simulink model "AE_BoltEV_LMDI"  (R2026a)
settings: Solver=ode23t  StartTime=0  StopTime=1800  FixedStep=Ts  MaxStep=0.01  EnableMultiTasking=on
InitFcn:
  | AE_BoltEV_LMDI_Params;
undefined symbols (not defined in the file): id_map, iq_map, Is_map, n_loss_bp, P, P_cu_map, P_iron_map, T_loss_bp, Tmax, V_oc
libraries: nesl_utility x14, fl_lib x12, autolibshared x2, sdl_lib x2, autolibmappedmotor x1, sl_discontinuities x1
(part 1 of 3)
CloseFcn:
  | try,close(h1_IPMSMTorqueBasedLoad),end
  | clear h1_IPMSMTorqueBasedLoad
  | 
  | clear simlog_IPMSMTorqueBasedLoad
  | clear logsout_IPMSMTorqueBasedLoad
Description:
  | IPMSM Torque-Based Load Control
settings Model: SimulationMode=accelerator  Creator=The MathWorks, Inc.  LastModifiedBy=fsk
settings DataIOCC: Decimation=100  MaxDataPoints=0  OutputTimes=0:0.1:1800  LoggingFileName=Results/paperA_sim_logsout.mat
settings SimscapeCC: SimscapeNormalizeSystem=off  SimscapeNominalValues="[{\"value\":\"1\",\"unit\":\"A\"},{\"value\":\"1\",\"unit\":\"bar\"},{\"value\":\"1\",\"unit\":\"cm^2\"},{\"value\":\"1\",\"unit\":\"cm^3/s\"},{\"value\":\"1\",\"unit\":\"kJ/kg\"},{\"value\":\"1\",\"unit\":\"kW\"},{\"value\":\"1\",\"unit\":\"l\"},{\"value\":\"1\",\"unit\":\"N\"},{\"value\":\"1\",\"unit\":\"N*m\"},{\"value\":\"1\",\"unit\":\"V\"}]"  SimscapeLogType=none  SimscapeLogSimulationStatistics=on  SimscapeLogToSDI=on  SimscapeLogName=simlog_TeslaBEV  SimscapeLogDecimation=50.0  SimscapeLogDataHistory=210000.0

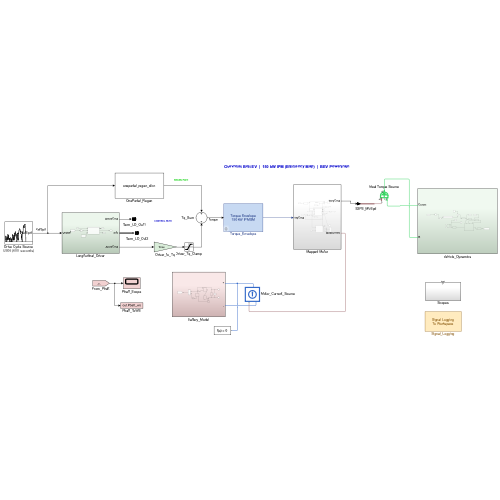
[thumbnail: Simulink's stored preview of the top-level diagram]
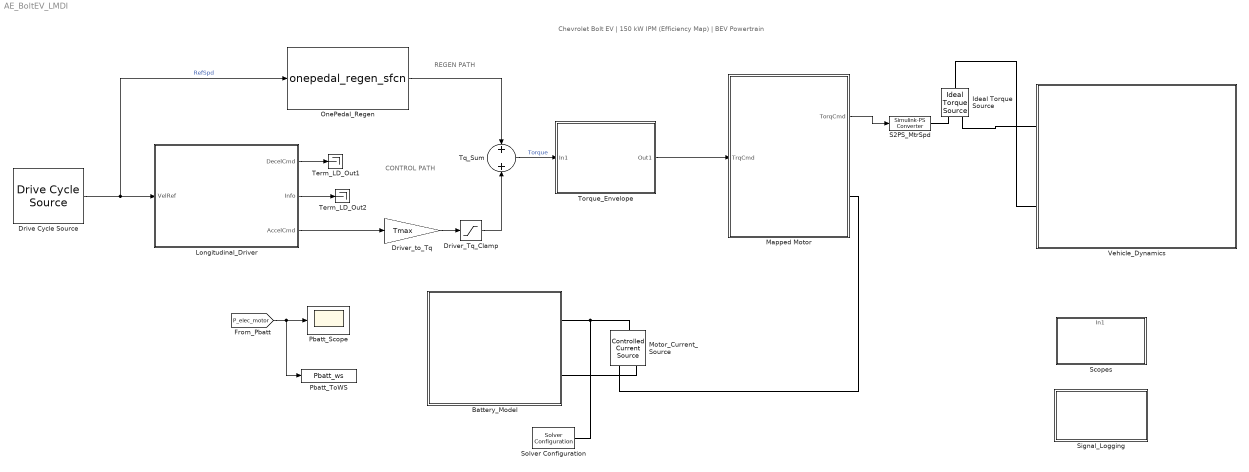
== system AE_BoltEV_LMDI ==
  note: Chevrolet Bolt EV | 150 kW IPM (Efficiency Map) | BEV Powertrain
  note: REGEN PATH
  note: CONTROL PATH
  Battery_Model : Subsystem
  Drive Cycle Source : autolibshared/Drive Cycle Source  cycleVar=WLTP Class 3  fileVar=cycleFTP75.mat  tfinal="1800  seconds"  cycleRepeat=off  outAccPort=off  outGearPort=off  gearList=No gear data  t_wot1=5  xdot_woto=0  xdot_wot1=140  t_wot2=20  xdot_wot2=0  t_wotend=30  srcUnit=m/s  outUnit=m/s  srcAccUnit=m/s/s  outAccUnit=m/s^2  dt=0  aMode=1  faultOption=off  velBnd=2  velBndUnit=mph  inUnit=m/s  timeBnd=1  failOption=off  stopSim=off  maxFaultCnt=10  maxFaultTime=2  maxTotFaultTime=15  traceOption=off  dtTrace=1  traceWindow=10  lastDCname=UDDS  lastOutUnit=mph  lastDT=0  lastTB=1  lastSB=2  forceCalcBound=off
  Driver_Tq_Clamp : Saturate  UpperLimit=inf  LowerLimit=0
  Driver_to_Tq : Gain  Gain=Tmax
  Ideal Torque Source : fl_lib/Mechanical/Mechanical Sources/Ideal Torque Source
  Longitudinal_Driver : Subsystem
  Mapped Motor : Subsystem
  Motor_Current_Source : fl_lib/Electrical/Electrical Sources/Controlled Current Source
  OnePedal_Regen : M-S-Function  FunctionName=onepedal_regen_sfcn
  Pbatt_Scope : Scope
      settings: ActiveDisplayYMinimum=-0.1838964776883894  ActiveDisplayYMaximum=2.2550682991955053
  Pbatt_ToWS : ToWorkspace  VariableName=Pbatt_ws  SampleTime=0.1
  S2PS_MtrSpd : nesl_utility/Simulink-PS Converter  PhysicalDomain=network_engine_domain  SubClassName=ps_input  LeftPortType=input  RightPortType=output  PseudoPeriodic=off  Frequencies=[]  NoiseDistribution=none  NoiseParameters=[]  Unit=N*m  AffineConversion=off  FilteringAndDerivatives=provide  SimscapeFilterOrder=1  InputFilterTimeConstant=0.001  UdotUserProvided=0
  Scopes : Subsystem
      settings: PortSchema="{\"entries\":[{\"content\":{\"sides\":[{\"content\":{},\"type\":\"ConnectorPlacement.EquallySpacedRectSide\",\"uuid\":\"17434833-391c-4e2f-b8de-edaf643e1441\"},{\"content\":{\"side\":\"RIGHT\"},\"type\":\"ConnectorPlacement.EquallySpacedRectSide\",\"uuid\":\"4cc327a6-11fd-412e-a651-a3b2a821325f\"},{\"content\":{\"connectorIds\":[\"In1\"],\"side\":\"TOP\"},\"type\":\"ConnectorPlacement.EquallySpacedRectSide\",\"uuid\":\"245fa48b-b588-4cde-bdc7-ab5c96e46538\"}]},\"type\":\"ConnectorPlacement.EquallySpacedConnector\",\"uuid\":\"adff8972-0810-4b2b-8c89-762b3a096b75\"}],\"packageUris\":[\"http://schema.mathworks.com/mf0/Connector/R2020b\"],\"version\":\"1.0\"}"
  Signal_Logging : Subsystem
      mask Display: disp('Signal Logging\nTo Workspace')
  Solver Configuration : nesl_utility/Solver Configuration  PhysicalDomain=network_engine_domain  SubClassName=solver  LeftPortType=input  RightPortType=generic  Tones=[]  Harmonics=[]  SimulateNoise=off  Profile=off  UseLocalSampling=off  EnableSwitchedLinearOptims=on  FrequencyDomain=off  UseCCode=off  RelTol=0.001  AbsTol=0.001  MinStep=1e-09  ToWorkspace=off  RevertToSquareIcSolve=off  NumHomotopyIterations=100  PhasorMode=off  PhasorModeNumHarmonics=1  ConsistencySolver=NEWTON_XTOL_AFTER_FTOL  CanonicalOrdering=CANONICAL  OptimizeIntermediates=OPTIMIZED  IndexReductionMethod=DerivativeReplacement  DoDC=off  ResidualTolerance=1e-09  ConsistencyTolSource=GLOBAL  ConsistencyAbsTol=0.001  ConsistencyRelTol=0.001  ConsistencyTolFactor=0.001  UseLocalSolver=off  LocalSolverChoice=NE_BACKWARD_EULER_ADVANCER  ResolveIndetEquations=on  FunctionEvalNumThread=1  LocalSolverSampleTime=0.001  DoFixedCost=off  MaxNonlinIter=3  MaxModeIter=2  ComputeImpulses=off  ImpulseIterations=2  LinearAlgebra=auto  LinearAlgebraNumThread=0  EquationFormulation=NE_TIME_EF  DelaysMemoryBudget=1024  AutomaticFiltering=on  FilteringTimeConstant=0.001  PartitionStorageMethod=AS_NEEDED  PartitionMemoryBudget=1024  PartitionMethod=ROBUST  MultibodyUseLocalSolver=off  MultibodyLocalSolverChoice=ODE1  MultibodyLocalSolverSampleTime=0.001
  Term_LD_Out1 : Terminator
  Term_LD_Out2 : Terminator
  Torque_Envelope : Subsystem
      mask DialogControl Control1 Prompt: (Add text here)
      mask DialogControl Control2 Prompt: (Add text here)
      mask Display: disp('Torque Envelope\n150 kW IPMSM')
  Tq_Sum : Sum
  Vehicle_Dynamics : Subsystem
  wires:
  Longitudinal_Driver/3(AccelCmd) -> Driver_to_Tq/1
  Tq_Sum/1 -> Torque_Envelope/1(In1)  "Torque"
  Driver_to_Tq/1 -> Driver_Tq_Clamp/1
  [P_elec_motor] -> Pbatt_Scope/1, Pbatt_ToWS/1
  Driver_Tq_Clamp/1 -> Tq_Sum/2
  Longitudinal_Driver/1(DecelCmd) -> Term_LD_Out1/1
  Longitudinal_Driver/2(Info) -> Term_LD_Out2/1
  Drive Cycle Source/1 -> OnePedal_Regen/1, Longitudinal_Driver/1(VelRef)  "RefSpd"
  OnePedal_Regen/1 -> Tq_Sum/1
  Torque_Envelope/1(Out1) -> Mapped Motor/1(TrqCmd)
  Mapped Motor/1(TorqCmd) -> S2PS_MtrSpd/1
  connections:
  Motor_Current_Source/RConn2 -- Battery_Model/RConn2
  Battery_Model/RConn1 -- Solver Configuration/RConn1 -- Motor_Current_Source/LConn1
  S2PS_MtrSpd/RConn1 -- Ideal Torque Source/RConn1
  Ideal Torque Source/LConn1 -- Vehicle_Dynamics/LConn2
  Vehicle_Dynamics/LConn1 -- Ideal Torque Source/RConn2
  Mapped Motor/RConn1 -- Motor_Current_Source/RConn1

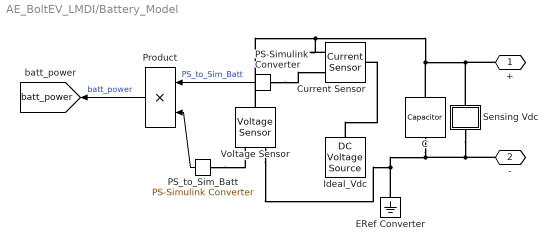
== system AE_BoltEV_LMDI/Battery_Model ==
  C : fl_lib/Electrical/Electrical Elements/Capacitor  c=Cdc F  r=1e-6 Ohm  g=0 1/Ohm  i_specify=off  i_priority=None  i=0 A  i_nominal_specify=off  i_nominal_value=1  i_nominal_unit=A  v_specify=off  v_priority=None  v=0 V  v_nominal_specify=off  v_nominal_value=1  v_nominal_unit=V  vc_specify=on  vc_priority=None  vc=Vnom V  vc_nominal_specify=off  vc_nominal_value=1  vc_nominal_unit=V
  Current Sensor : fl_lib/Electrical/Electrical Sensors/Current Sensor
  ERef Converter : fl_lib/Electrical/Electrical Elements/Electrical Reference
  Ideal_Vdc : fl_lib/Electrical/Electrical Sources/DC Voltage Source  v0=350 V
  PS-Simulink Converter : nesl_utility/PS-Simulink Converter  PhysicalDomain=network_engine_domain  SubClassName=ps_output  LeftPortType=input  RightPortType=output  PseudoPeriodic=off  Frequencies=[]  VectorFormat=inherit  Unit=A  AffineConversion=off
  PS_to_Sim_Batt : nesl_utility/PS-Simulink Converter  PhysicalDomain=network_engine_domain  SubClassName=ps_output  LeftPortType=input  RightPortType=output  PseudoPeriodic=off  Frequencies=[]  VectorFormat=inherit  Unit=V  AffineConversion=off
  Product : Product
  Sensing Vdc : Subsystem
      mask Display: disp('vdc')
  Voltage Sensor : fl_lib/Electrical/Electrical Sensors/Voltage Sensor
  + : PMIOPort  Side=Right
  - : PMIOPort  Port=2  Side=Right
  tag scope: batt_power=global
  wires:
  PS_to_Sim_Batt/1 -> Product/2
  Product/1 -> [batt_power]  "batt_power"
  PS-Simulink Converter/1 -> Product/1  "PS_to_Sim_Batt"
  connections:
  Voltage Sensor/LConn1 -- Current Sensor/RConn2 -- C/LConn1 -- +/RConn1 -- Sensing Vdc/LConn1
  PS-Simulink Converter/LConn1 -- Current Sensor/RConn1
  PS_to_Sim_Batt/LConn1 -- Voltage Sensor/RConn1
  -/RConn1 -- Sensing Vdc/RConn1 -- ERef Converter/LConn1 -- Voltage Sensor/RConn2 -- C/RConn1
  Ideal_Vdc/LConn1 -- Current Sensor/LConn1

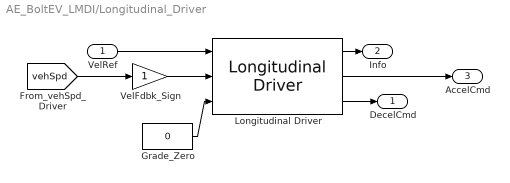
== system AE_BoltEV_LMDI/Longitudinal_Driver ==
  VelRef : Inport
  Grade_Zero : Constant  Value=0
  Longitudinal Driver : autolibshared/Longitudinal Driver  extAccelOvr=off  extDecelOvr=off  extAccelHld=off  extDecelHld=off  extAccelZero=off  extDecelZero=off  cntrlType=PI  shftType=None  velUnits=m/s  gearOut=off  Kp=400  Ki=80  Kff=0.15  Kg=.01  VehVelVec=[0 15 30 100]  KffVec=[.1 .1]  KpVec=[400 400 200 200]  KiVec=[80 80 40 40]  KgVec=[0 0]  m=1928  Kpt=3000  tau=.1  L=2  aR=126  bR=0  cR=0.4336  g=9.81  vnom=100  Kaw=5  tauerr=.03  tauPt=0.2  GearInit=0  tShift=.1  pdlVec=[0.1 0.4 0.5 0.9]  upShftTbl=[-1 12.9375 26.4375 39.9375 51.18749999999999 62.4375 72.84375 83.25;-1 16.3125 29.8125 43.3125 54.5624 65.8125 76.78125 87.75;-1 19.6875 33.1875 46.68749999999999 57.9375 69.1875 80.71875 92.25;-1 33 52.5 77.25 100.5 138.75 161.875 185]  dwnShftTbl=[1 9.5625 23.0625 36.5625 47.8125 59.0625 68.90625 78.75;1 12.9375 26.4375 39.9375 51.18749999999999 62.4375 72.84375 83.25;1 16.3125 29.8125 43.3125 54.562499 65.8125 76.78125 87.75;1 19.6875 33.1875 46.68749999999999 57.9375 69.1875 80.71875 92.25]  tClutch=.5  tRev=.5  tPark=120  aMode=2  UpGearVec="[0  1  2  3  4  5  6  7]"  DownGearVec="[1  2  3  4  5  6  7  8]"
  VelFdbk_Sign : Gain
  DecelCmd : Outport
  Info : Outport  Port=2
  AccelCmd : Outport  Port=3
  wires:
  VelRef/1 -> Longitudinal Driver/1
  [vehSpd] -> VelFdbk_Sign/1
  Longitudinal Driver/2 -> AccelCmd/1
  Longitudinal Driver/1 -> Info/1
  Grade_Zero/1 -> Longitudinal Driver/3
  Longitudinal Driver/3 -> DecelCmd/1
  VelFdbk_Sign/1 -> Longitudinal Driver/2
